simulink model "atrias_boom_nmStand_fullCtrl"  (R2015a)
settings: Solver=ode23t  StartTime=0.0  StopTime=t_end  FixedStep=0.001  MaxStep=1e-3  RelTol=1e-3
InitFcn:
  | addpath('../common/')
  | colors
StartFcn:
  | tic
StopFcn:
  | %stopscript
values from neighbouring files (symbols this model uses):
  A1_notch_f1 = -2*cos(fnotch_f1*sample_time)    [set_control_params.m]
  A2_notch_f1 = 1    [set_control_params.m]
  A_lpf_dtau = 1 + B1_lpf_dtau + B2_lpf_dtau    [set_control_params.m]
  ankle_stiffness = 1/2*pi    (= 1.57079632679)    [mechanical_params.m]
  B1_lpf_dtau = -2*exp(-lpf_damping*fcut_dtau*sample_time)*cos(fcut_dtau*sample_time*sqrt(1-lpf_damping^2))    [set_control_params.m]
  B1_notch_f1 = -2*exp(-notch_damping*fnotch_f1*sample_time)*cos(fnotch_f1*sample_time*sqrt(1-notch_damping^2))    [set_control_params.m]
  B2_lpf_dtau = exp(-2*lpf_damping*fcut_dtau*sample_time)    [set_control_params.m]
  B2_notch_f1 = exp(-2*notch_damping*fnotch_f1*sample_time)    [set_control_params.m]
  b_hmotor = 0    [mechanical_params.m]
  b_leg_spring = 0.075*sqrt(k_leg_spring*0.5*.25^2)    [mechanical_params.m]
  b_rotor = 0*60/(2*pi)*9.725e-5    (= 0)    [mechanical_params.m]
  boom_mount_to_center_diagonal = boom_mount_to_center / cos(pitch_mount_angle)    [mechanical_params.m]    (also in set_control_params.m)
  breakaway_friction = [25 25 25 25]    [mechanical_params.m]
  contactThr = 0.35    [set_control_params.m]
  coulomb_friction = [20 20 20 20]    [mechanical_params.m]
  d_com = (d_hip_com_to_torso_com*m_torso)/(m_torso + num_legs*m_hshaft)    [mechanical_params.m]
  delta_phi_max = 160*pi/180    (= 2.79252680319)    [mechanical_params.m]    (also in set_control_params.m)
  delta_phi_max_buffer = 20*pi/180    (= 0.349065850399)    [set_control_params.m]
  delta_phi_max_dropoff = 2*pi/180    (= 0.0349065850399)    [set_control_params.m]
  delta_phi_min = 25.5*pi/180    (= 0.445058959259)    [mechanical_params.m]    (also in set_control_params.m)
  friction_linear_zone = [0.5 0.5 0.5 0.5].*pi/180    [mechanical_params.m]
  g = 9.803    [mechanical_params.m]    (also in set_control_params.m = 9.81)
  gain_nodes_sea_torque = [0,65,350,700]    [set_control_params.m]
  HIP_MTR_MAX_CONT_TORQUE = HIP_MTR_MAX_CONT_CURRENT*HIP_MOTOR_CONSTANT*HIP_MTR_GEAR_RATIO    (= 86.0016)    [set_control_params.m]
  HIP_MTR_MAX_TORQUE = max_current_hip*Kt_hip*N_h    (= 629.28)    [mechanical_params.m]
  initial_boom_pitch = 0    [mechanical_params.m]
  initial_boom_roll = asin((initial_com_height + boom_mount_to_com + boom_mount_to_center*tan(pitch_mount_angle) - (base_12(2) + yshaft_12(2))) / (l_boom + boom_mount_to_center_diagonal))    [mechanical_params.m]
  initial_boom_yaw = 0    [mechanical_params.m]
  initial_hip_roll = 0*pi/180    (= 0)    [mechanical_params.m]
  initial_winch_angle = -12 * pi/180    (= -0.209439510239)    [mechanical_params.m]
  k_gn = m_total*g/0.01    (= 57041.421916)    [mechanical_params.m]
  k_gt = m_total*g/0.1    (= 5704.1421916)    [mechanical_params.m]
  k_leg_spring = 4118.3    [mechanical_params.m]    (also in set_control_params.m)
  K_notch_f1 = (1+B1_notch_f1+B2_notch_f1)/(1+A1_notch_f1+A2_notch_f1)    [set_control_params.m]
  k_phi = 5000    [mechanical_params.m]
  k_sea = [4118.3 4118.3 4118.3 4118.3]    [set_control_params.m]
  Kb_leg = 0.121    [mechanical_params.m]
  kd_boom_roll_Ctrl = 0    [main_1_nmStand.m]    (also in main_2_nmStand_moveBoom.m)
  kd_lateral = 2*sqrt(kp_lateral*0.8)    [set_control_params.m]
  kd_shin_max = kd_pd_avoid_limits    (= 1000)    [set_control_params.m]
  kd_shin_min = kd_pd_avoid_limits    (= 1000)    [set_control_params.m]
  kd_splay_max = kd_pd_avoid_limits    (= 1000)    [set_control_params.m]
  kd_splay_min = kd_pd_avoid_limits    (= 1000)    [set_control_params.m]
  kd_thigh_max = kd_pd_avoid_limits    (= 1000)    [set_control_params.m]
  kd_thigh_min = kd_pd_avoid_limits    (= 1000)    [set_control_params.m]
  kd_winch = td_winch*kp_winch    (= 989.239577798)    [mechanical_params.m]
  kp_boom_roll_Ctrl = 0    [main_1_nmStand.m]    (also in main_2_nmStand_moveBoom.m)
  kp_lateral = 1000    [set_control_params.m]
  kp_sea_torque = [0.3, 0.3, 6.0, 6.0]    [set_control_params.m]
  kp_shin_max = kp_pd_avoid_limits    (= 5000)    [set_control_params.m]
  kp_shin_min = kp_pd_avoid_limits    (= 5000)    [set_control_params.m]
  kp_splay_max = kp_pd_avoid_limits    (= 5000)    [set_control_params.m]
  kp_splay_min = kp_pd_avoid_limits/10    (= 500)    [set_control_params.m]
  kp_thigh_max = kp_pd_avoid_limits    (= 5000)    [set_control_params.m]
  kp_thigh_min = kp_pd_avoid_limits    (= 5000)    [set_control_params.m]
  kp_winch = winch_gravity_comp/(3*pi/180)    (= 19784.791556)    [mechanical_params.m]
  Kt_leg = 0.121    [mechanical_params.m]
  l_boom = 1.8161    [mechanical_params.m]    (also in set_control_params.m)
  L_leg = 0.102e-3    (= 0.000102)    [mechanical_params.m]
  l_seg = 0.5    [mechanical_params.m]    (also in set_control_params.m)
  l_v = l_seg*cos(min_splay_angle/2)    [set_control_params.m]
  lateral_offset = 0.2    [set_control_params.m]
  lateral_target_angle_right = -6*pi/180    (= -0.10471975512)    [set_control_params.m]
  lateral_transition_force = 150    [set_control_params.m]
  LEG_MTR_MAX_TORQUE = max_current_leg * Kt_leg * N    (= 1210)    [mechanical_params.m]
  loaded_unloaded_torque_threshold = 65*ones(1,4)    [set_control_params.m]
  lowerleg_12 = 0.40    (= 0.4)    [mechanical_params.m]
  m_boom = 4.49    [mechanical_params.m]
  m_fblink = 0.46    [mechanical_params.m]    (also in set_control_params.m)
  m_foot = 0.0857    [mechanical_params.m]
  m_hshaft = 18    [mechanical_params.m]    (also in set_control_params.m = 20)
  m_leg = m_thigh + m_lowerleg + m_shin + m_fblink    (= 2.3438)    [mechanical_params.m]
  m_leg_motor = 18    [set_control_params.m]
  m_lowerleg = 0.4438    [mechanical_params.m]    (also in set_control_params.m)
  m_output_gear = 1e-5    (= 1e-05)    [mechanical_params.m]    (also in set_control_params.m)
  m_rotor = 1e-5    (= 1e-05)    [mechanical_params.m]    (also in set_control_params.m)
  m_shin = 0.75    [mechanical_params.m]    (also in set_control_params.m)
  m_thigh = 0.69    [mechanical_params.m]    (also in set_control_params.m)
  m_torso = 17.5    [mechanical_params.m]    (also in set_control_params.m = 17.9)
  m_total = num_legs*(m_hshaft + m_thigh + m_lowerleg + m_shin + m_fblink + 2*m_gearing) + m_torso    (= 58.18772)    [mechanical_params.m]    (also in set_control_params.m = 62.58772)
  m_virtual_gear = 1e-5    (= 1e-05)    [mechanical_params.m]    (also in set_control_params.m)
  m_yshaft = 12.89    [mechanical_params.m]
  max_current_leg = 200    [mechanical_params.m]
  max_sagittal_loaded_torque = 833    [set_control_params.m]
  max_sagittal_unloaded_torque = 267    [set_control_params.m]
  max_torque_lateral = min(MTR_HIP_MAX_CURRENT, HIP_CURRENT_LIMIT)*HIP_MOTOR_CONSTANT*HIP_MTR_GEAR_RATIO    [set_control_params.m]
  max_voltage_leg = 50    [mechanical_params.m]
  maximum_lateral_angle = 18*pi/180    (= 0.314159265359)    [set_control_params.m]
  min_splay_angle = 45*pi/180    (= 0.785398163397)    [set_control_params.m]
  min_splay_buffer = 1*pi/180    (= 0.0174532925199)    [set_control_params.m]
  min_splay_dropoff = 5*pi/180    (= 0.0872664625997)    [set_control_params.m]
  minimum_lateral_angle = -9.5*pi/180    (= -0.165806278939)    [set_control_params.m]
  mu_hmotor = 0.90    (= 0.9)    [mechanical_params.m]
  mu_motor = 0.85    [mechanical_params.m]
  mu_slide = 0.8    [mechanical_params.m]
  mu_stick = 0.9    [mechanical_params.m]
  N = 50    [mechanical_params.m]
  N_h = r_hip_shaft / r_hip_gearhead    (= 57)    [mechanical_params.m]
  phi_max_collision = -5*pi/180    (= -0.0872664625997)    [mechanical_params.m]
  phi_roll_max = pi + 16*pi/180    (= 3.42084533391)    [mechanical_params.m]
  phi_roll_min = pi - 9*pi/180    (= 2.98451302091)    [mechanical_params.m]
  phi_shin_max = 3*pi/2 + 17.5*pi/180    (= 5.01782159948)    [mechanical_params.m]    (also in set_control_params.m)
  phi_shin_max_buffer = 20*pi/180    (= 0.349065850399)    [set_control_params.m]
  phi_shin_max_dropoff = 2*pi/180    (= 0.0349065850399)    [set_control_params.m]
  phi_shin_min = pi - 45*pi/180    (= 2.35619449019)    [mechanical_params.m]    (also in set_control_params.m)
  phi_shin_min_buffer = 20*pi/180    (= 0.349065850399)    [set_control_params.m]
  phi_shin_min_dropoff = 2*pi/180    (= 0.0349065850399)    [set_control_params.m]
  phi_thigh_max = pi + 45*pi/180    (= 3.92699081699)    [mechanical_params.m]    (also in set_control_params.m)
  phi_thigh_max_buffer = 20*pi/180    (= 0.349065850399)    [set_control_params.m]
  phi_thigh_max_dropoff = 2*pi/180    (= 0.0349065850399)    [set_control_params.m]
  phi_thigh_min = pi/2 - 17.5*pi/180    (= 1.2653637077)    [mechanical_params.m]    (also in set_control_params.m)
  phi_thigh_min_buffer = 20*pi/180    (= 0.349065850399)    [set_control_params.m]
  phi_thigh_min_dropoff = 2*pi/180    (= 0.0349065850399)    [set_control_params.m]
  r_hip_gearhead = 0.009525    [mechanical_params.m]
  r_hip_shaft = 0.542925    [mechanical_params.m]
  R_leg = 0.052    [mechanical_params.m]
  r_rotor = 0.001    [mechanical_params.m]
  r_virtual_gear = N*r_rotor    (= 0.05)    [mechanical_params.m]
  releaseThr = 0.2    [set_control_params.m]
  sample_time = 0.001    [set_control_params.m]
  ... (+19 more)
undefined symbols (not defined in the file or in its folder): A_lpf_velocity, B1_lpf_velocity, B2_lpf_velocity, base_color_d, boom_color_d, c, c_jointstop, CtrlPar_theta0, eref, fblink_color_d, floor_color_d, FmaxBFSH, FmaxGLU, FmaxHAM, FmaxHFL, FmaxRF, FmaxVAS, foot_color_d, FPCtrlPar, hshaft_color_d, j_motor, K, lateral_motor_efficiency, LLCtrlPar, loptBFSH, loptGLU, loptHAM, loptHFL, loptRF, loptVAS, lowerleg_color_d, lslackBFSH, lslackGLU, lslackHAM, lslackHFL, lslackRF, lslackVAS, MidDelay_discrete, Newton, output_sample_time, phi12_max, phi12_min, phi23_max, phi23_min, phimaxRFk, phimaxVAS, phirefBFSH, phirefGLU, phirefHAMh, phirefHAMk, phirefHFL, phirefRFh, phirefRFk, phirefVAS, phiScaleRFk, phiScaleVAS, rad ... (+40)
libraries: sm_lib x210, nesl_utility x140, simulink x58, simulink_extras x26, fl_lib x16, mblibv1 x2, commnoisgen2 x1
(part 13 of 19)

== system atrias_boom_nmStand_fullCtrl/Control/Behavior Control/Virtual Neuromuscular Control/Muscle Layer/L Knee Joint Limits ==
  note: Knee Joint Limits
  phi [rad]1 : Inport
  dphi [rad/s]1 : Inport  Port=2
  Constant : Constant  Value=0
  Gain1 : Gain  Gain=c_jointstop
  Gain5 : Gain  Gain=-1
  Gain6 : Gain  Gain=c_jointstop
  Gain7 : Gain  Gain=1/w_max_jointstop
  Manual Switch : ManualSwitch
  Mux1 : Mux  Inputs=2
  Mux2 : Mux  Inputs=2
  Overextension Torque1 : Fcn  Expr="- u(1)  *  (1-u(2)) * (u(2)<1) * (u(1)>0)"
  Overflexion Torque : Fcn  Expr="- u(1)  *  (1-u(2)) * (u(2)<1) * (u(1)<0)"
  Sum1 : Sum  Inputs=|+-
  Sum2 : Sum  Inputs=|+-
  Sum3 : Sum
  overextension angle1 : Constant  Value=phi12_max
  overflexion angle : Constant  Value=phi12_min
  M_stop [Nm]1 : Outport
  wires:
  Mux2/1 -> Overextension Torque1/1
  Gain6/1 -> Mux2/1
  dphi [rad/s]1/1 -> Gain7/1
  overextension angle1/1 -> Sum1/2
  phi [rad]1/1 -> Sum1/1, Sum2/1
  Sum1/1 -> Gain6/1
  Gain7/1 -> Gain5/1, Mux1/2
  Gain1/1 -> Mux1/1
  Sum2/1 -> Gain1/1
  overflexion angle/1 -> Sum2/2
  Mux1/1 -> Overflexion Torque/1
  Gain5/1 -> Mux2/2
  Overflexion Torque/1 -> Sum3/2
  Overextension Torque1/1 -> Sum3/1
  Sum3/1 -> Manual Switch/1
  Constant/1 -> Manual Switch/2
  Manual Switch/1 -> M_stop [Nm]1/1

== system atrias_boom_nmStand_fullCtrl/Control/Behavior Control/Virtual Neuromuscular Control/Muscle Layer/L Knee Joint Limits1 ==
  note: Knee Joint Limits
  phi [rad]1 : Inport
  dphi [rad/s]1 : Inport  Port=2
  Constant : Constant  Value=0
  Gain1 : Gain  Gain=c_jointstop
  Gain5 : Gain  Gain=-1
  Gain6 : Gain  Gain=c_jointstop
  Gain7 : Gain  Gain=1/w_max_jointstop
  Manual Switch : ManualSwitch
  Mux1 : Mux  Inputs=2
  Mux2 : Mux  Inputs=2
  Overextension Torque1 : Fcn  Expr="- u(1)  *  (1-u(2)) * (u(2)<1) * (u(1)>0)"
  Overflexion Torque : Fcn  Expr="- u(1)  *  (1-u(2)) * (u(2)<1) * (u(1)<0)"
  Sum1 : Sum  Inputs=|+-
  Sum2 : Sum  Inputs=|+-
  Sum3 : Sum
  overextension angle1 : Constant  Value=phi12_max
  overflexion angle : Constant  Value=phi12_min
  M_stop [Nm]1 : Outport
  wires:
  Mux2/1 -> Overextension Torque1/1
  Gain6/1 -> Mux2/1
  dphi [rad/s]1/1 -> Gain7/1
  overextension angle1/1 -> Sum1/2
  phi [rad]1/1 -> Sum1/1, Sum2/1
  Sum1/1 -> Gain6/1
  Gain7/1 -> Gain5/1, Mux1/2
  Gain1/1 -> Mux1/1
  Sum2/1 -> Gain1/1
  overflexion angle/1 -> Sum2/2
  Mux1/1 -> Overflexion Torque/1
  Gain5/1 -> Mux2/2
  Overflexion Torque/1 -> Sum3/2
  Overextension Torque1/1 -> Sum3/1
  Sum3/1 -> Manual Switch/1
  Constant/1 -> Manual Switch/2
  Manual Switch/1 -> M_stop [Nm]1/1

== system atrias_boom_nmStand_fullCtrl/Control/Behavior Control/Virtual Neuromuscular Control/Muscle Layer/RF ==
  note: Rectus Femoris Muscle-Tendon Dynamics
  note: Excitation Contraction Coupling
  STIM : Inport
  lmtc [m] : Inport  Port=2
  1 : Product  Inputs=**  SaturateOnIntegerOverflow=on  InputSameDT=on  OutDataTypeStr=Inherit: Same as first input
  1/lslack : Gain  Gain=1/lslackRF  SaturateOnIntegerOverflow=on  OutDataTypeStr=Inherit: Same as input  ParamDataTypeStr=Inherit: Same as input
  BE force-length relation : Subsystem
  CE force-length relation : Subsystem
  CE inverse force-velocity relation : Subsystem
  Constant : Constant  Value=lslackRF
  ECC TransferFcn : simulink_extras/Additional Linear/Transfer Fcn (with initial outputs)  N=[1]  D="[tau  1]"  Y0=preA  U0=0
      settings: AttributesFormatString=pre-activation: %<Y0>
  Fmax : Gain  Gain=FmaxRF  SaturateOnIntegerOverflow=on  OutDataTypeStr=Inherit: Same as input  ParamDataTypeStr=Inherit: Same as input
  Fv = Fse / (A*Fce) : Product  Inputs=*/  SaturateOnIntegerOverflow=on  InputSameDT=on  OutDataTypeStr=Inherit: Same as first input
  Integrator : Integrator  InitialConditionSource=external  LowerSaturationLimit=0.05
  PE force-length relation : Subsystem
  SE force-length relation : Subsystem
  Saturation : Saturate  UpperLimit=1  LowerLimit=0.01
  Sum : Sum  Inputs=|+-  SaturateOnIntegerOverflow=on  InputSameDT=on  OutDataTypeStr=Inherit: Same as first input
  Sum2 : Sum  Inputs=|-+  SaturateOnIntegerOverflow=on  InputSameDT=on  OutDataTypeStr=Inherit: Same as first input
  Sum3 : Sum  SaturateOnIntegerOverflow=on  InputSameDT=on  OutDataTypeStr=Inherit: Same as first input
  Sum4 : Sum  SaturateOnIntegerOverflow=on  InputSameDT=on  OutDataTypeStr=Inherit: Same as first input
  lce/lopt : Gain  Gain=1/loptRF  SaturateOnIntegerOverflow=on  OutDataTypeStr=Inherit: Same as input  ParamDataTypeStr=Inherit: Same as input
  vmax*lopt : Gain  Gain=vmaxRF*loptRF  SaturateOnIntegerOverflow=on  OutDataTypeStr=Inherit: Same as input  ParamDataTypeStr=Inherit: Same as input
  Fmtc : Outport  InitialOutput=0
  Lce : Outport  Port=2  InitialOutput=0
  Vce : Outport  Port=3  InitialOutput=0
  A : Outport  Port=4  InitialOutput=0
  wires:
  Integrator/1 -> Sum/2, lce/lopt/1, Lce/1  "lce"
  Sum/1 -> 1/lslack/1  "lse"
  lce/lopt/1 -> CE force-length relation/1(lce [lopt]), BE force-length relation/1(lce [lopt]), PE force-length relation/1(lce [lopt])
  Fv = Fse / (A*Fce)/1 -> CE inverse force-velocity relation/1(Fv[Fmax])  "fv"
  vmax*lopt/1 -> Integrator/1, Vce/1  "vce"
  lmtc [m]/1 -> Sum2/2, Sum/1  "lmtc"
  Fmax/1 -> Fmtc/1  "Fmtc"
  1/lslack/1 -> SE force-length relation/1(lse [lslack])
  SE force-length relation/1(fse [Fmax]) -> Fmax/1, Sum4/1
  Sum2/1 -> Integrator/2
  Constant/1 -> Sum2/1
  CE force-length relation/1(fce [Fmax]) -> 1/1
  Sum4/1 -> Fv = Fse / (A*Fce)/1
  PE force-length relation/1(fpe [Fmax]) -> Sum3/1
  1/1 -> Sum3/2
  BE force-length relation/1(fbe [Fmax]) -> Sum4/2
  Sum3/1 -> Fv = Fse / (A*Fce)/2
  CE inverse force-velocity relation/1(v[vmax]) -> vmax*lopt/1
  STIM/1 -> ECC TransferFcn/1
  ECC TransferFcn/1 -> Saturation/1
  Saturation/1 -> 1/2, A/1

== system atrias_boom_nmStand_fullCtrl/Control/Behavior Control/Virtual Neuromuscular Control/Muscle Layer/RF Link ==
  note: RF Attachment
  phi34 [rad] : Inport
  phi23 [rad] : Inport  Port=2
  Constant1 : Constant  Value=phimaxRFk
  Constant2 : Constant  Value=phirefRFk
  Constant3 : Constant  Value=rRFh
  Constant4 : Constant  Value=lslackRF+loptRF
  Constant5 : Constant  Value=phirefRFh
  Demux : Demux  Outputs=2
  Display : Display
  Gain1 : Gain  Gain=rRFkmax
  Gain2 : Gain  Gain=rhoRFh
  Gain3 : Gain  Gain=phiScaleRFk
  Gain4 : Gain  Gain=rhoRFk/phiScaleRFk
  Gain5 : Gain  Gain=phiScaleRFk
  Mux : Mux  Inputs=2
  Product : Product  RndMeth=Zero
  Sum1 : Sum  Inputs=-+
  Sum2 : Sum  Inputs=|+-
  Sum3 : Sum  Inputs=-+|
  Sum4 : Sum  Inputs=|+-
  Sum5 : Sum  Inputs=++-
  length change term : Trigonometry
  offset correction term : Trigonometry
  variable lever term : Trigonometry  Operator=cos
  lmtu [m] : Outport
  lever34 [m] : Outport  Port=2
  lever23 [m] : Outport  Port=3
  wires:
  Sum5/1 -> Display/1, lmtu [m]/1
  Constant4/1 -> Sum5/2
  Gain4/1 -> Sum5/3
  Gain2/1 -> Sum5/1
  phi34 [rad]/1 -> Sum4/1
  Constant5/1 -> Sum4/2
  Sum4/1 -> Product/1
  Constant3/1 -> Product/2, lever34 [m]/1
  Product/1 -> Gain2/1
  phi23 [rad]/1 -> Sum3/2
  Sum3/1 -> Gain3/1
  Constant1/1 -> Sum3/1, Sum2/2
  Sum2/1 -> Gain5/1
  Constant2/1 -> Sum2/1
  length change term/1 -> Sum1/2
  offset correction term/1 -> Sum1/1
  Sum1/1 -> Mux/1
  variable lever term/1 -> Mux/2
  Mux/1 -> Gain1/1
  Gain1/1 -> Demux/1
  Demux/2 -> lever23 [m]/1
  Demux/1 -> Gain4/1
  Gain3/1 -> variable lever term/1, length change term/1
  Gain5/1 -> offset correction term/1

== system atrias_boom_nmStand_fullCtrl/Control/Behavior Control/Virtual Neuromuscular Control/Muscle Layer/RF Link1 ==
  note: RF Attachment
  phi34 [rad] : Inport
  phi23 [rad] : Inport  Port=2
  Constant1 : Constant  Value=phimaxRFk
  Constant2 : Constant  Value=phirefRFk
  Constant3 : Constant  Value=rRFh
  Constant4 : Constant  Value=lslackRF+loptRF
  Constant5 : Constant  Value=phirefRFh
  Demux : Demux  Outputs=2
  Gain1 : Gain  Gain=rRFkmax
  Gain2 : Gain  Gain=rhoRFh
  Gain3 : Gain  Gain=phiScaleRFk
  Gain4 : Gain  Gain=rhoRFk/phiScaleRFk
  Gain5 : Gain  Gain=phiScaleRFk
  Mux : Mux  Inputs=2
  Product : Product  RndMeth=Zero
  Sum1 : Sum  Inputs=-+
  Sum2 : Sum  Inputs=|+-
  Sum3 : Sum  Inputs=-+|
  Sum4 : Sum  Inputs=|+-
  Sum5 : Sum  Inputs=++-
  length change term : Trigonometry
  offset correction term : Trigonometry
  variable lever term : Trigonometry  Operator=cos
  lmtu [m] : Outport
  lever34 [m] : Outport  Port=2
  lever23 [m] : Outport  Port=3
  wires:
  Sum5/1 -> lmtu [m]/1
  Constant4/1 -> Sum5/2
  Gain4/1 -> Sum5/3
  Gain2/1 -> Sum5/1
  phi34 [rad]/1 -> Sum4/1
  Constant5/1 -> Sum4/2
  Sum4/1 -> Product/1
  Constant3/1 -> Product/2, lever34 [m]/1
  Product/1 -> Gain2/1
  phi23 [rad]/1 -> Sum3/2
  Sum3/1 -> Gain3/1
  Constant1/1 -> Sum3/1, Sum2/2
  Sum2/1 -> Gain5/1
  Constant2/1 -> Sum2/1
  length change term/1 -> Sum1/2
  offset correction term/1 -> Sum1/1
  Sum1/1 -> Mux/1
  variable lever term/1 -> Mux/2
  Mux/1 -> Gain1/1
  Gain1/1 -> Demux/1
  Demux/2 -> lever23 [m]/1
  Demux/1 -> Gain4/1
  Gain3/1 -> variable lever term/1, length change term/1
  Gain5/1 -> offset correction term/1

== system atrias_boom_nmStand_fullCtrl/Control/Behavior Control/Virtual Neuromuscular Control/Muscle Layer/RF1 ==
  note: Rectus Femoris Muscle-Tendon Dynamics
  note: Excitation Contraction Coupling
  STIM : Inport
  lmtc [m] : Inport  Port=2
  1 : Product  Inputs=**  SaturateOnIntegerOverflow=on  InputSameDT=on  OutDataTypeStr=Inherit: Same as first input
  1/lslack : Gain  Gain=1/lslackRF  SaturateOnIntegerOverflow=on  OutDataTypeStr=Inherit: Same as input  ParamDataTypeStr=Inherit: Same as input
  BE force-length relation : Subsystem
  CE force-length relation : Subsystem
  CE inverse force-velocity relation : Subsystem
  Constant : Constant  Value=lslackRF
  ECC TransferFcn : simulink_extras/Additional Linear/Transfer Fcn (with initial outputs)  N=[1]  D="[tau  1]"  Y0=preA  U0=0
      settings: AttributesFormatString=pre-activation: %<Y0>
  Fmax : Gain  Gain=FmaxRF  SaturateOnIntegerOverflow=on  OutDataTypeStr=Inherit: Same as input  ParamDataTypeStr=Inherit: Same as input
  Fv = Fse / (A*Fce) : Product  Inputs=*/  SaturateOnIntegerOverflow=on  InputSameDT=on  OutDataTypeStr=Inherit: Same as first input
  Integrator : Integrator  InitialConditionSource=external  LowerSaturationLimit=0.05
  PE force-length relation : Subsystem
  SE force-length relation : Subsystem
  Saturation : Saturate  UpperLimit=1  LowerLimit=0.01
  Sum : Sum  Inputs=|+-  SaturateOnIntegerOverflow=on  InputSameDT=on  OutDataTypeStr=Inherit: Same as first input
  Sum2 : Sum  Inputs=|-+  SaturateOnIntegerOverflow=on  InputSameDT=on  OutDataTypeStr=Inherit: Same as first input
  Sum3 : Sum  SaturateOnIntegerOverflow=on  InputSameDT=on  OutDataTypeStr=Inherit: Same as first input
  Sum4 : Sum  SaturateOnIntegerOverflow=on  InputSameDT=on  OutDataTypeStr=Inherit: Same as first input
  lce/lopt : Gain  Gain=1/loptRF  SaturateOnIntegerOverflow=on  OutDataTypeStr=Inherit: Same as input  ParamDataTypeStr=Inherit: Same as input
  vmax*lopt : Gain  Gain=vmaxRF*loptRF  SaturateOnIntegerOverflow=on  OutDataTypeStr=Inherit: Same as input  ParamDataTypeStr=Inherit: Same as input
  Fmtc : Outport  InitialOutput=0
  Lce : Outport  Port=2  InitialOutput=0
  Vce : Outport  Port=3  InitialOutput=0
  A : Outport  Port=4  InitialOutput=0
  wires:
  Integrator/1 -> Sum/2, lce/lopt/1, Lce/1  "lce"
  Sum/1 -> 1/lslack/1  "lse"
  lce/lopt/1 -> CE force-length relation/1(lce [lopt]), BE force-length relation/1(lce [lopt]), PE force-length relation/1(lce [lopt])
  Fv = Fse / (A*Fce)/1 -> CE inverse force-velocity relation/1(Fv[Fmax])  "fv"
  vmax*lopt/1 -> Integrator/1, Vce/1  "vce"
  lmtc [m]/1 -> Sum2/2, Sum/1  "lmtc"
  Fmax/1 -> Fmtc/1  "Fmtc"
  1/lslack/1 -> SE force-length relation/1(lse [lslack])
  SE force-length relation/1(fse [Fmax]) -> Fmax/1, Sum4/1
  Sum2/1 -> Integrator/2
  Constant/1 -> Sum2/1
  CE force-length relation/1(fce [Fmax]) -> 1/1
  Sum4/1 -> Fv = Fse / (A*Fce)/1
  PE force-length relation/1(fpe [Fmax]) -> Sum3/1
  1/1 -> Sum3/2
  BE force-length relation/1(fbe [Fmax]) -> Sum4/2
  Sum3/1 -> Fv = Fse / (A*Fce)/2
  CE inverse force-velocity relation/1(v[vmax]) -> vmax*lopt/1
  STIM/1 -> ECC TransferFcn/1
  ECC TransferFcn/1 -> Saturation/1
  Saturation/1 -> 1/2, A/1

== system atrias_boom_nmStand_fullCtrl/Control/Behavior Control/Virtual Neuromuscular Control/Muscle Layer/VAS ==
  note: VASTI Muscle-Tendon Dynamics
  note: Excitation Contraction Coupling
  STIM : Inport
  lmtc [m] : Inport  Port=2
  1 : Product  Inputs=**  SaturateOnIntegerOverflow=on  InputSameDT=on  OutDataTypeStr=Inherit: Same as first input
  1/lslack : Gain  Gain=1/lslackVAS  SaturateOnIntegerOverflow=on  OutDataTypeStr=Inherit: Same as input  ParamDataTypeStr=Inherit: Same as input
  BE force-length relation : Subsystem
  CE force-length relation : Subsystem
  CE inverse force-velocity relation : Subsystem
  Constant : Constant  Value=lslackVAS
  ECC TransferFcn : simulink_extras/Additional Linear/Transfer Fcn (with initial outputs)  N=[1]  D="[tau  1]"  Y0=preA  U0=0
      settings: AttributesFormatString=pre-activation: %<Y0>
  Fmax : Gain  Gain=FmaxVAS  SaturateOnIntegerOverflow=on  OutDataTypeStr=Inherit: Same as input  ParamDataTypeStr=Inherit: Same as input
  Fv = Fse / (A*Fce) : Product  Inputs=*/  SaturateOnIntegerOverflow=on  InputSameDT=on  OutDataTypeStr=Inherit: Same as first input
  Integrator : Integrator  InitialConditionSource=external  LowerSaturationLimit=0.05
  PE force-length relation : Subsystem
  SE force-length relation : Subsystem
  Saturation : Saturate  UpperLimit=1  LowerLimit=0.01
  Sum : Sum  Inputs=|+-  SaturateOnIntegerOverflow=on  InputSameDT=on  OutDataTypeStr=Inherit: Same as first input
  Sum2 : Sum  Inputs=|-+  SaturateOnIntegerOverflow=on  InputSameDT=on  OutDataTypeStr=Inherit: Same as first input
  Sum3 : Sum  SaturateOnIntegerOverflow=on  InputSameDT=on  OutDataTypeStr=Inherit: Same as first input
  Sum4 : Sum  SaturateOnIntegerOverflow=on  InputSameDT=on  OutDataTypeStr=Inherit: Same as first input
  lce/lopt : Gain  Gain=1/loptVAS  SaturateOnIntegerOverflow=on  OutDataTypeStr=Inherit: Same as input  ParamDataTypeStr=Inherit: Same as input
  vmax*lopt : Gain  Gain=vmaxVAS*loptVAS  SaturateOnIntegerOverflow=on  OutDataTypeStr=Inherit: Same as input  ParamDataTypeStr=Inherit: Same as input
  Fmtc : Outport  InitialOutput=0
  Lce : Outport  Port=2  InitialOutput=0
  Vce : Outport  Port=3  InitialOutput=0
  A : Outport  Port=4  InitialOutput=0
  wires:
  Integrator/1 -> Sum/2, lce/lopt/1, Lce/1  "lce"
  Sum/1 -> 1/lslack/1  "lse"
  lce/lopt/1 -> CE force-length relation/1(lce [lopt]), BE force-length relation/1(lce [lopt]), PE force-length relation/1(lce [lopt])
  Fv = Fse / (A*Fce)/1 -> CE inverse force-velocity relation/1(Fv[Fmax])  "fv"
  vmax*lopt/1 -> Integrator/1, Vce/1  "vce"
  lmtc [m]/1 -> Sum2/2, Sum/1  "lmtc"
  Fmax/1 -> Fmtc/1  "Fmtc"
  1/lslack/1 -> SE force-length relation/1(lse [lslack])
  SE force-length relation/1(fse [Fmax]) -> Fmax/1, Sum4/1
  Sum2/1 -> Integrator/2
  Constant/1 -> Sum2/1
  CE force-length relation/1(fce [Fmax]) -> 1/1
  Sum4/1 -> Fv = Fse / (A*Fce)/1
  PE force-length relation/1(fpe [Fmax]) -> Sum3/1
  1/1 -> Sum3/2
  BE force-length relation/1(fbe [Fmax]) -> Sum4/2
  Sum3/1 -> Fv = Fse / (A*Fce)/2
  CE inverse force-velocity relation/1(v[vmax]) -> vmax*lopt/1
  STIM/1 -> ECC TransferFcn/1
  ECC TransferFcn/1 -> Saturation/1
  Saturation/1 -> 1/2, A/1

== system atrias_boom_nmStand_fullCtrl/Control/Behavior Control/Virtual Neuromuscular Control/Muscle Layer/VAS Link ==
  note: Muscle Length and Moment Arm
  phi23 [rad] : Inport
  Constant : Constant  Value=lslackVAS+loptVAS
  Constant1 : Constant  Value=phimaxVAS
  Constant2 : Constant  Value=phirefVAS
  Demux : Demux  Outputs=2
  Gain1 : Gain  Gain=rVASmax
  Gain3 : Gain  Gain=phiScaleVAS
  Gain4 : Gain  Gain=rhoVAS/phiScaleVAS
  Gain5 : Gain  Gain=phiScaleVAS
  Mux : Mux  Inputs=2
  Sum1 : Sum  Inputs=-+
  Sum2 : Sum  Inputs=|+-
  Sum3 : Sum  Inputs=-+|
  Sum5 : Sum  Inputs=|+-
  length change term : Trigonometry
  offset correction term : Trigonometry
  variable lever term : Trigonometry  Operator=cos
  lmtu [m] : Outport
  lever [m] : Outport  Port=2
  wires:
  Constant/1 -> Sum5/1
  Sum5/1 -> lmtu [m]/1
  phi23 [rad]/1 -> Sum3/2
  Sum3/1 -> Gain3/1
  Constant1/1 -> Sum3/1, Sum2/2
  Sum2/1 -> Gain5/1
  Constant2/1 -> Sum2/1
  length change term/1 -> Sum1/2
  offset correction term/1 -> Sum1/1
  Sum1/1 -> Mux/1
  variable lever term/1 -> Mux/2
  Mux/1 -> Gain1/1
  Gain1/1 -> Demux/1
  Demux/2 -> lever [m]/1
  Demux/1 -> Gain4/1
  Gain3/1 -> variable lever term/1, length change term/1
  Gain5/1 -> offset correction term/1
  Gain4/1 -> Sum5/2

== system atrias_boom_nmStand_fullCtrl/Control/Behavior Control/Virtual Neuromuscular Control/Muscle Layer/VAS Link1 ==
  note: Muscle Length and Moment Arm
  phi23 [rad] : Inport
  Constant : Constant  Value=lslackVAS+loptVAS
  Constant1 : Constant  Value=phimaxVAS
  Constant2 : Constant  Value=phirefVAS
  Demux : Demux  Outputs=2
  Gain1 : Gain  Gain=rVASmax
  Gain3 : Gain  Gain=phiScaleVAS
  Gain4 : Gain  Gain=rhoVAS/phiScaleVAS
  Gain5 : Gain  Gain=phiScaleVAS
  Mux : Mux  Inputs=2
  Sum1 : Sum  Inputs=-+
  Sum2 : Sum  Inputs=|+-
  Sum3 : Sum  Inputs=-+|
  Sum5 : Sum  Inputs=|+-
  length change term : Trigonometry
  offset correction term : Trigonometry
  variable lever term : Trigonometry  Operator=cos
  lmtu [m] : Outport
  lever [m] : Outport  Port=2
  wires:
  Constant/1 -> Sum5/1
  Sum5/1 -> lmtu [m]/1
  phi23 [rad]/1 -> Sum3/2
  Sum3/1 -> Gain3/1
  Constant1/1 -> Sum3/1, Sum2/2
  Sum2/1 -> Gain5/1
  Constant2/1 -> Sum2/1
  length change term/1 -> Sum1/2
  offset correction term/1 -> Sum1/1
  Sum1/1 -> Mux/1
  variable lever term/1 -> Mux/2
  Mux/1 -> Gain1/1
  Gain1/1 -> Demux/1
  Demux/2 -> lever [m]/1
  Demux/1 -> Gain4/1
  Gain3/1 -> variable lever term/1, length change term/1
  Gain5/1 -> offset correction term/1
  Gain4/1 -> Sum5/2

== system atrias_boom_nmStand_fullCtrl/Control/Behavior Control/Virtual Neuromuscular Control/Muscle Layer/VAS1 ==
  note: VASTI Muscle-Tendon Dynamics
  note: Excitation Contraction Coupling
  STIM : Inport
  lmtc [m] : Inport  Port=2
  1 : Product  Inputs=**  SaturateOnIntegerOverflow=on  InputSameDT=on  OutDataTypeStr=Inherit: Same as first input
  1/lslack : Gain  Gain=1/lslackVAS  SaturateOnIntegerOverflow=on  OutDataTypeStr=Inherit: Same as input  ParamDataTypeStr=Inherit: Same as input
  BE force-length relation : Subsystem
  CE force-length relation : Subsystem
  CE inverse force-velocity relation : Subsystem
  Constant : Constant  Value=lslackVAS
  ECC TransferFcn : simulink_extras/Additional Linear/Transfer Fcn (with initial outputs)  N=[1]  D="[tau  1]"  Y0=preA  U0=0
      settings: AttributesFormatString=pre-activation: %<Y0>
  Fmax : Gain  Gain=FmaxVAS  SaturateOnIntegerOverflow=on  OutDataTypeStr=Inherit: Same as input  ParamDataTypeStr=Inherit: Same as input
  Fv = Fse / (A*Fce) : Product  Inputs=*/  SaturateOnIntegerOverflow=on  InputSameDT=on  OutDataTypeStr=Inherit: Same as first input
  Integrator : Integrator  InitialConditionSource=external  LowerSaturationLimit=0.05
  PE force-length relation : Subsystem
  SE force-length relation : Subsystem
  Saturation : Saturate  UpperLimit=1  LowerLimit=0.01
  Sum : Sum  Inputs=|+-  SaturateOnIntegerOverflow=on  InputSameDT=on  OutDataTypeStr=Inherit: Same as first input
  Sum2 : Sum  Inputs=|-+  SaturateOnIntegerOverflow=on  InputSameDT=on  OutDataTypeStr=Inherit: Same as first input
  Sum3 : Sum  SaturateOnIntegerOverflow=on  InputSameDT=on  OutDataTypeStr=Inherit: Same as first input
  Sum4 : Sum  SaturateOnIntegerOverflow=on  InputSameDT=on  OutDataTypeStr=Inherit: Same as first input
  lce/lopt : Gain  Gain=1/loptVAS  SaturateOnIntegerOverflow=on  OutDataTypeStr=Inherit: Same as input  ParamDataTypeStr=Inherit: Same as input
  vmax*lopt : Gain  Gain=vmaxVAS*loptVAS  SaturateOnIntegerOverflow=on  OutDataTypeStr=Inherit: Same as input  ParamDataTypeStr=Inherit: Same as input
  Fmtc : Outport  InitialOutput=0
  Lce : Outport  Port=2  InitialOutput=0
  Vce : Outport  Port=3  InitialOutput=0
  A : Outport  Port=4  InitialOutput=0
  wires:
  Integrator/1 -> Sum/2, lce/lopt/1, Lce/1  "lce"
  Sum/1 -> 1/lslack/1  "lse"
  lce/lopt/1 -> CE force-length relation/1(lce [lopt]), BE force-length relation/1(lce [lopt]), PE force-length relation/1(lce [lopt])
  Fv = Fse / (A*Fce)/1 -> CE inverse force-velocity relation/1(Fv[Fmax])  "fv"
  vmax*lopt/1 -> Integrator/1, Vce/1  "vce"
  lmtc [m]/1 -> Sum2/2, Sum/1  "lmtc"
  Fmax/1 -> Fmtc/1  "Fmtc"
  1/lslack/1 -> SE force-length relation/1(lse [lslack])
  SE force-length relation/1(fse [Fmax]) -> Fmax/1, Sum4/1
  Sum2/1 -> Integrator/2
  Constant/1 -> Sum2/1
  CE force-length relation/1(fce [Fmax]) -> 1/1
  Sum4/1 -> Fv = Fse / (A*Fce)/1
  PE force-length relation/1(fpe [Fmax]) -> Sum3/1
  1/1 -> Sum3/2
  BE force-length relation/1(fbe [Fmax]) -> Sum4/2
  Sum3/1 -> Fv = Fse / (A*Fce)/2
  CE inverse force-velocity relation/1(v[vmax]) -> vmax*lopt/1
  STIM/1 -> ECC TransferFcn/1
  ECC TransferFcn/1 -> Saturation/1
  Saturation/1 -> 1/2, A/1

== system atrias_boom_nmStand_fullCtrl/Control/Behavior Control/Virtual Neuromuscular Control/Neural Control Layer/L Stance Phase (sagittal) ==
  note: M4: compensate swing leg
  note: M3: balance trunk
  note: M2: prevent knee overextension
  note: M1: realize compliant leg
  note: 0: Prestimulations
  note: Left Stance Phase Control
  CtrlPar : Inport
  theta_tgt [rad] : Inport  Port=2
  theta dtheta [rad rad/s] : Inport  Port=3
  CStim_HSw : Inport  Port=4
  FmVAS : Inport  Port=5
  LceBFSH : Inport  Port=6
  Enable : EnablePort  StatesWhenEnabling=reset  ZeroCross=off
  Demux1 : Demux  Outputs=5
  Demux2 : Demux
  Demux4 : Demux  Outputs=6
  Demux5 : Demux  Outputs=5
  Demux7 : Demux  Outputs=2
  Divide{4..6,8..9,12..13,15,17,19..22} (13 alike) : Product
  Gain : Gain  Gain=-1
  Gain2 : Gain  Gain=-1
  Gain3 : Gain  Gain=-1
  Mux1 : Mux  Inputs=3
  Mux2 : Mux  Inputs=2
  Mux3 : Mux  Inputs=3
  Sum1 : Sum  Inputs=-+|  SaturateOnIntegerOverflow=on  InputSameDT=on  OutDataTypeStr=Inherit: Same as first input
  Sum{2,7..8,11} (4 alike) : Sum  Inputs=|++  SaturateOnIntegerOverflow=on  InputSameDT=on  OutDataTypeStr=Inherit: Same as first input
  Sum3 : Sum  Inputs=-+|  SaturateOnIntegerOverflow=on  InputSameDT=on  OutDataTypeStr=Inherit: Same as first input
  Sum4 : Sum  Inputs=-+|  SaturateOnIntegerOverflow=on  InputSameDT=on  OutDataTypeStr=Inherit: Same as first input
  Terminator : Terminator
  Terminator1 : Terminator
  parStPreS : Selector  InputPortWidth=St_i  Indices=parSt_PreS_i
  parSt_M1 : Selector  InputPortWidth=St_i  Indices=parSt_M1_i
  parSt_M2 : Selector  InputPortWidth=St_i  Indices=parSt_M2_i
  parSt_M3 : Selector  InputPortWidth=St_i  Indices=parSt_M3_i
  parSt_M4 : Selector  InputPortWidth=St_i  Indices=parSt_M4_i
  positive half{1..4,6} (5 alike) : Saturate  UpperLimit=inf  LowerLimit=0  ZeroCross=off
  S_St_0 : Outport  OutputWhenDisabled=reset  InitialOutput=0
  S_M1 [VAS] : Outport  Port=2  OutputWhenDisabled=reset  InitialOutput=0
  S_M2 [VAS BFSH] : Outport  Port=3  OutputWhenDisabled=reset  InitialOutput=0
  S_M3 [HFL GLU HAM] : Outport  Port=4  OutputWhenDisabled=reset  InitialOutput=0
  S_M4 [HFL GLU HAM] : Outport  Port=5  OutputWhenDisabled=reset  InitialOutput=0
  wires:
  Demux4/6 -> Terminator1/1
  Demux4/5 -> Terminator/1
  Divide9/1 -> Sum11/2
  Sum11/1 -> Divide21/1, Mux3/2  "GLU"
  Divide12/1 -> Sum11/1
  Divide17/1 -> Sum7/2
  Sum7/1 -> Mux3/1  "HFL"
  Divide22/1 -> Sum7/1
  Demux1/4 -> Divide9/1  "SGainCRF_GLU"
  Demux1/2 -> Divide17/1  "SGainCHAM_HFL"
  Demux4/4 -> Divide9/2  "Stim_CRF"
  Demux4/3 -> Divide17/2  "Stim_CHAM"
  Divide21/1 -> Mux3/3  "HAM"
  Demux1/5 -> Divide21/2  "SGainGLU_HAM"
  Mux3/1 -> S_M4 [HFL GLU HAM]/1
  Demux4/2 -> Divide22/2  "Stim_CGLU"
  Demux4/1 -> Divide12/2  "Stim_CHFL"
  CStim_HSw/1 -> Demux4/1
  Demux1/3 -> Divide12/1  "SGainCHFL_GLU"
  Demux1/1 -> Divide22/1  "SGainCGLU_HFL"
  parSt_M4/1 -> Demux1/1
  positive half6/1 -> Mux1/3
  positive half2/1 -> Mux1/2
  positive half1/1 -> Mux1/1
  theta_tgt [rad]/1 -> Sum1/1
  Divide6/1 -> positive half6/1  "HAM"
  Demux5/5 -> Divide6/2  "SGainGLU_HAM"
  Mux1/1 -> S_M3 [HFL GLU HAM]/1
  Sum8/1 -> positive half2/1, Divide6/1  "GLU"
  Sum2/1 -> positive half1/1  "HFL"
  Divide5/1 -> Sum8/2
  Divide4/1 -> Sum8/1
  Divide20/1 -> Sum2/2
  Divide19/1 -> Sum2/1
  Gain3/1 -> Divide20/1
  Gain2/1 -> Divide19/1
  Sum1/1 -> Divide4/1, Gain2/1
  Demux7/2 -> Divide5/1, Gain3/1  "dtheta"
  Demux7/1 -> Sum1/2  "theta"
  theta dtheta [rad rad/s]/1 -> Demux7/1
  Demux5/4 -> Divide5/2  "GainDTh_GLU"
  Demux5/3 -> Divide4/2  "GainTh_GLU"
  Demux5/2 -> Divide20/2  "GainDTh_HFL"
  Demux5/1 -> Divide19/2  "GainTh_HFL"
  parSt_M3/1 -> Demux5/1
  Mux2/1 -> S_M2 [VAS BFSH]/1
  LceBFSH/1 -> Sum4/2, Sum3/2
  Demux2/3 -> Sum4/1  "loff_BFSH"
  positive half4/1 -> Divide13/1
  Sum4/1 -> positive half4/1
  Gain/1 -> Mux2/1  "VAS"
  Divide13/1 -> Mux2/2  "BFSH"
  Divide15/1 -> Gain/1
  Demux2/1 -> Sum3/1  "loff_BFSH_VAS"
  positive half3/1 -> Divide15/1
  Demux2/4 -> Divide13/2  "LGain_BFSH"
  Demux2/2 -> Divide15/2  "LGainBFSH_VAS"
  Sum3/1 -> positive half3/1
  parSt_M2/1 -> Demux2/1
  FmVAS/1 -> Divide8/2
  Divide8/1 -> S_M1 [VAS]/1  "VAS"
  parSt_M1/1 -> Divide8/1  "FGain_VAS"
  parStPreS/1 -> S_St_0/1
  CtrlPar/1 -> parSt_M1/1, parSt_M2/1, parSt_M4/1, parSt_M3/1, parStPreS/1

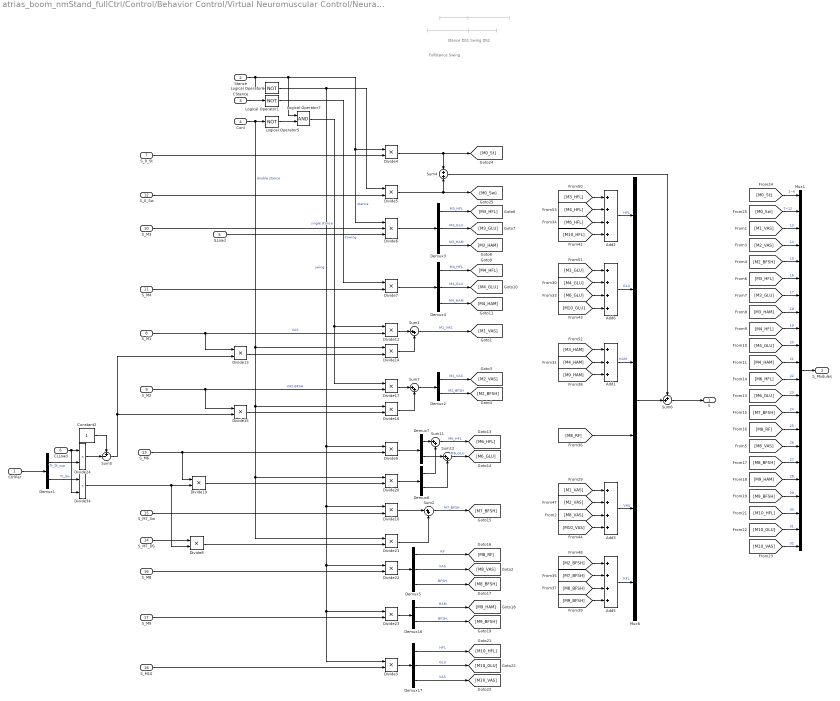
== system atrias_boom_nmStand_fullCtrl/Control/Behavior Control/Virtual Neuromuscular Control/Neural Control Layer/L Stance, Swing, Trans (sagittal) ==
  note: |--------------------|------------------------------|
  note: |------------------------------|--------------------|
  note: FullStance Swing
  note: Stance DS1 Swing DS2
  CtrlPar : Inport
  Stance : Inport  Port=2
  CStance : Inport  Port=3
  ConI : Inport  Port=4
  ILLoad : Inport  Port=5
  CLLoad : Inport  Port=6
  S_0_St : Inport  Port=7
  S_M1 : Inport  Port=8
  S_M2 : Inport  Port=9
  S_M3 : Inport  Port=10
  S_M4 : Inport  Port=11
  S_0_Sw : Inport  Port=12
  S_M6 : Inport  Port=13
  S_M7_DS : Inport  Port=14
  S_M7_Sw : Inport  Port=15
  S_M8 : Inport  Port=16
  S_M9 : Inport  Port=17
  S_M10 : Inport  Port=18
  Add1 : Sum  Inputs=3
  Add{2..3,5..6} (4 alike) : Sum  Inputs=4
  Constant2 : Constant
  Demux{1..2,6..7,16} (5 alike) : Demux  Outputs=2
  Demux{3..5,17} (4 alike) : Demux  Outputs=3
  Divide{3..5,7..10,12..17,19..24,34} (20 alike) : Product
  Divide6 : Product  Inputs=3
  Logical Operator1 : Logic  Operator=NOT  AllPortsSameDT=off  OutDataTypeStr=boolean
  Logical Operator5 : Logic  Operator=NOT  AllPortsSameDT=off  OutDataTypeStr=boolean
  Logical Operator6 : Logic  Operator=NOT  AllPortsSameDT=off  OutDataTypeStr=boolean
  Logical Operator7 : Logic  AllPortsSameDT=off  OutDataTypeStr=boolean
  Mux1 : Mux  Inputs=22
  Mux6 : Mux  Inputs=6
  Sum{1..2,7,11..12} (5 alike) : Sum  Inputs=|++  SaturateOnIntegerOverflow=on  InputSameDT=on  OutDataTypeStr=Inherit: Same as first input
  Sum4 : Sum  SaturateOnIntegerOverflow=on  InputSameDT=on  OutDataTypeStr=Inherit: Same as first input
  Sum5 : Sum  Inputs=+-|  SaturateOnIntegerOverflow=on  InputSameDT=on  OutDataTypeStr=Inherit: Same as first input
  Sum6 : Sum  Inputs=++|  SaturateOnIntegerOverflow=on  InputSameDT=on  OutDataTypeStr=Inherit: Same as first input
  S : Outport  OutputWhenDisabled=reset  InitialOutput=0
  S_Modules : Outport  Port=2  OutputWhenDisabled=reset  InitialOutput=0
  wires:
  Mux1/1 -> S_Modules/1
  [M0_Sw] -> Mux1/2  "7~12"
  [M0_St] -> Mux1/1  "1~6"
  [M1_VAS] -> Mux1/3  "13"
  [M2_BFSH] -> Mux1/5  "15"
  [M2_VAS] -> Mux1/4  "14"
  [M6_GLU] -> Mux1/13  "23"
  [M6_HFL] -> Mux1/12  "22"
  [M4_HAM] -> Mux1/11  "21"
  [M4_GLU] -> Mux1/10  "20"
  [M4_HFL] -> Mux1/9  "19"
  [M3_HAM] -> Mux1/8  "18"
  [M3_GLU] -> Mux1/7  "17"
  [M3_HFL] -> Mux1/6  "16"
  [M10_VAS] -> Add3/4
  [M10_HFL] -> Add2/4
  [M9_HAM] -> Add1/3
  [M8_RF] -> Mux6/4
  [M8_BFSH] -> Add5/3
  [M9_BFSH] -> Add5/4
  [M7_BFSH] -> Add5/2
  [M6_HFL] -> Add2/3
  [M4_HAM] -> Add1/2
  [M4_HFL] -> Add2/2
  [M3_HAM] -> Add1/1
  [M3_HFL] -> Add2/1
  [M2_BFSH] -> Add5/1
  [M2_VAS] -> Add3/2
  [M1_VAS] -> Add3/1
  [M10_GLU] -> Add6/4
  [M6_GLU] -> Add6/3
  [M4_GLU] -> Add6/2
  [M3_GLU] -> Add6/1
  Demux17/3 -> [M10_VAS]  "VAS"
  Demux17/2 -> [M10_GLU]  "GLU"
  Demux17/1 -> [M10_HFL]  "HFL"
  Demux16/2 -> [M9_BFSH]  "BFSH"
  Demux16/1 -> [M9_HAM]  "HAM"
  Divide3/1 -> Demux17/1
  S_M10/1 -> Divide3/2
  Divide23/1 -> Demux16/1
  S_M9/1 -> Divide23/2
  Divide22/1 -> Demux5/1
  S_M8/1 -> Divide22/2
  Sum2/1 -> [M7_BFSH]  "M7_BFSH"
  S_M7_DS/1 -> Divide8/1
  Divide8/1 -> Divide21/2
  S_M7_Sw/1 -> Divide10/2
  Sum5/1 -> Divide15/2, Divide13/2
  Divide21/1 -> Sum2/2
  Sum12/1 -> [M6_GLU]  "M6_GLU"
  Sum11/1 -> [M6_HFL]  "M6_HFL"
  Divide19/1 -> Divide20/2
  Demux7/1 -> Sum11/1
  Demux6/2 -> Sum12/2
  Demux6/1 -> Sum11/2
  Divide20/1 -> Demux6/1
  Demux7/2 -> Sum12/1
  Divide9/1 -> Demux7/1
  S_M6/1 -> Divide19/1, Divide9/2
  Demux3/3 -> [M3_HAM]  "M3_HAM"
  Demux3/2 -> [M3_GLU]  "M3_GLU"
  Demux3/1 -> [M3_HFL]  "M3_HFL"
  Divide6/1 -> Demux3/1
  ILLoad/1 -> Divide6/3
  S_M3/1 -> Divide6/2
  Demux2/2 -> [M2_BFSH]  "M2_BFSH"
  Demux2/1 -> [M2_VAS]  "M2_VAS"
  Sum7/1 -> Demux2/1
  Divide17/1 -> Sum7/1
  S_M2/1 -> Divide15/1, Divide17/2  "VAS BFSH"
  Sum1/1 -> [M1_VAS]  "M1_VAS"
  Divide15/1 -> Divide16/2
  Divide16/1 -> Sum7/2
  Divide14/1 -> Sum1/2
  Divide13/1 -> Divide14/2
  Divide12/1 -> Sum1/1
  S_M1/1 -> Divide13/1, Divide12/2  "VAS"
  Divide4/1 -> [M0_St], Sum4/1
  Divide5/1 -> Sum4/2, [M0_Sw]
  S_0_St/1 -> Divide4/2
  S_0_Sw/1 -> Divide5/2
  Sum4/1 -> Sum6/1
  Sum6/1 -> S/1
  Mux6/1 -> Sum6/2
  Logical Operator6/1 -> Divide22/1, Divide23/1, Divide3/1, Divide10/1, Divide9/1, Divide5/1  "swing"
  Divide34/1 -> Divide8/2, Divide19/2
  Logical Operator7/1 -> Divide17/1, Divide12/1  "single stance"
  Divide7/1 -> Demux4/1
  Demux1/2 -> Divide34/1  "Tr_Sw"
  Add5/1 -> Mux6/6  "KFL"
  Add3/1 -> Mux6/5  "VAS"
  Demux4/3 -> [M4_HAM]  "M4_HAM"
  Add1/1 -> Mux6/3  "HAM"
  Demux4/2 -> [M4_GLU]  "M4_GLU"
  Add6/1 -> Mux6/2  "GLU"
  Add2/1 -> Mux6/1  "HFL"
  Demux4/1 -> [M4_HFL]  "M4_HFL"
  CLLoad/1 -> Divide34/2, Divide24/1
  Constant2/1 -> Sum5/1
  Divide24/1 -> Sum5/2
  Demux1/1 -> Divide24/2  "Tr_St_sup"
  Logical Operator1/1 -> Divide7/1  "Cswing"
  CStance/1 -> Logical Operator1/1
  S_M4/1 -> Divide7/2
  Logical Operator5/1 -> Logical Operator7/2
  ConI/1 -> Divide14/1, Divide16/1, Divide21/1, Divide20/1, Logical Operator5/1  "double stance"
  Stance/1 -> Divide6/1, Divide4/1, Logical Operator7/1, Logical Operator6/1  "stance"
  CtrlPar/1 -> Demux1/1
  [M8_VAS] -> Add3/3
  [M10_GLU] -> Mux1/21  "31"
  [M10_HFL] -> Mux1/20  "30"
  [M9_BFSH] -> Mux1/19  "29"
  [M9_HAM] -> Mux1/18  "28"
  [M8_BFSH] -> Mux1/17  "27"
  [M8_VAS] -> Mux1/16  "26"
  [M8_RF] -> Mux1/15  "25"
  [M7_BFSH] -> Mux1/14  "24"
  [M10_VAS] -> Mux1/22  "32"
  Divide10/1 -> Sum2/1
  Demux5/1 -> [M8_RF]  "RF"
  Demux5/3 -> [M8_BFSH]  "BFSH"
  Demux5/2 -> [M8_VAS]  "VAS"

== system atrias_boom_nmStand_fullCtrl/Control/Behavior Control/Virtual Neuromuscular Control/Neural Control Layer/L Swing Phase (sagittal) ==
  note: M10: prepare stance
  note: M9: stop leg
  note: M8: hold knee
  note: M7: flex knee
  note: M6: swing hip
  note: 0: Prestimulations
  note: Control During Stance -> Swing
  note: Left Swing Phase Control
  CtrlPar : Inport
  Stance : Inport  Port=2
  a_tgt : Inport  Port=3
  a : Inport  Port=4
  da : Inport  Port=5
  phiH : Inport  Port=6
  phiK : Inport  Port=7
  dphiK : Inport  Port=8
  l_clr : Inport  Port=9
  l : Inport  Port=10
  Enable : EnablePort  StatesWhenEnabling=reset
  Constant1 : Constant  Value=0  OutDataTypeStr=boolean
  Demux1 : Demux
  Divide{2..3,5,7..8} (5 alike) : Product
  Gain : Gain  Gain=-1
  Gain1 : Gain  Gain=-1
  Gain2 : Gain  Gain=-1
  Logical Operator : Logic  Operator=NOT  AllPortsSameDT=off  OutDataTypeStr=boolean
  Logical Operator1 : Logic  AllPortsSameDT=off  OutDataTypeStr=boolean
  Logical Operator2 : Logic  Operator=NOT  AllPortsSameDT=off  OutDataTypeStr=boolean
  Mux : Mux  Inputs=2
  Mux1 : Mux  Inputs=3
  Mux2 : Mux  Inputs=2
  Mux3 : Mux  Inputs=3
  Mux4 : Mux  Inputs=2
  Relational Operator : RelationalOperator  Operator=<=  OutDataTypeStr=boolean
  S-R Flip-Flop : simulink_extras/Flip Flops/S-R Flip-Flop  initial_condition=0
  Sum11 : Sum  Inputs=-+|  SaturateOnIntegerOverflow=on  InputSameDT=on  OutDataTypeStr=Inherit: Same as first input
  Sum6 : Sum  Inputs=|++  SaturateOnIntegerOverflow=on  InputSameDT=on  OutDataTypeStr=Inherit: Same as first input
  Sum7 : Sum  Inputs=|++  SaturateOnIntegerOverflow=on  InputSameDT=on  OutDataTypeStr=Inherit: Same as first input
  Terminator : Terminator
  kneei_flexion from alpha : Subsystem  TreatAsAtomicUnit=on
  kneeii_damp and hold &kneeiii_leg stop &kneeiv_stance preparation : Subsystem  TreatAsAtomicUnit=on
  negative half : Saturate  UpperLimit=0  LowerLimit=-inf  ZeroCross=off
  negative half2 : Saturate  UpperLimit=0  LowerLimit=-inf  ZeroCross=off
  negative half3 : Saturate  UpperLimit=0  LowerLimit=-inf  ZeroCross=off
  parSwH : Selector  InputPortWidth=Sw_i  Indices=parSwH_i
  parSwKi : Selector  InputPortWidth=Sw_i  Indices=parSwKi_i
  parSwPreS : Selector  InputPortWidth=Sw_i  Indices=parSwPreS_i
  positive half1 : Saturate  UpperLimit=inf  LowerLimit=0  ZeroCross=off
  positive half2 : Saturate  UpperLimit=inf  LowerLimit=0  ZeroCross=off
  S_Sw_0 : Outport  OutputWhenDisabled=reset  InitialOutput=0
  S_M6 [HFL GLU] : Outport  Port=2  OutputWhenDisabled=reset  InitialOutput=0
  S_M7_DS [BFSH] : Outport  Port=3  OutputWhenDisabled=reset  InitialOutput=0
  S_M7_Sw [VAS BFSH] : Outport  Port=4  OutputWhenDisabled=reset  InitialOutput=0
  M8 [RF VAS BFSH] : Outport  Port=5  OutputWhenDisabled=reset  InitialOutput=0
  M9 [HAM BFSH] : Outport  Port=6  OutputWhenDisabled=reset  InitialOutput=0
  M10 [HFL GLU VAS] : Outport  Port=7  OutputWhenDisabled=reset  InitialOutput=0
  Phase [M7 M8 M9 M10] : Outport  Port=8  OutputWhenDisabled=reset  InitialOutput=0
  wires:
  phiH/1 -> kneeii_damp and hold &kneeiii_leg stop &kneeiv_stance preparation/5(phiH)
  phiK/1 -> kneeii_damp and hold &kneeiii_leg stop &kneeiv_stance preparation/6(phiK)
  dphiK/1 -> kneeii_damp and hold &kneeiii_leg stop &kneeiv_stance preparation/7(dphiK)
  Gain2/1 -> negative half2/1
  da/1 -> kneeii_damp and hold &kneeiii_leg stop &kneeiv_stance preparation/4(da), negative half3/1, Gain2/1, negative half/1
  l_clr/1 -> Relational Operator/2
  l/1 -> Relational Operator/1
  Sum11/1 -> Gain/1, positive half2/1  "del_alp"
  a/1 -> Sum11/2, kneeii_damp and hold &kneeiii_leg stop &kneeiv_stance preparation/3(a)
  kneeii_damp and hold &kneeiii_leg stop &kneeiv_stance preparation/1(phase [M8 M9 M10]) -> Mux/2
  Mux/1 -> Phase [M7 M8 M9 M10]/1
  Divide8/1 -> Sum7/2
  Sum7/1 -> Mux2/2  "GLU"
  Divide2/1 -> Sum7/1  "GLU"
  negative half2/1 -> Divide8/2
  negative half3/1 -> Divide7/2
  Sum6/1 -> Mux2/1  "HFL"
  Divide7/1 -> Sum6/2
  Divide5/1 -> Sum6/1  "HFL"
  Demux1/4 -> Divide8/1  "Sw_dalpGain_GLU"
  Demux1/2 -> Divide7/1  "Sw_dalpGain_HFL"
  Mux1/1 -> M10 [HFL GLU VAS]/1
  Mux4/1 -> M9 [HAM BFSH]/1
  Mux3/1 -> M8 [RF VAS BFSH]/1
  Mux2/1 -> S_M6 [HFL GLU]/1
  kneeii_damp and hold &kneeiii_leg stop &kneeiv_stance preparation/9(SVAS_Sw_kiv) -> Mux1/3  "VAS"
  kneeii_damp and hold &kneeiii_leg stop &kneeiv_stance preparation/5(SHAM_Sw_kiii) -> Mux4/1  "HAM"
  parSwPreS/1 -> S_Sw_0/1
  Logical Operator2/1 -> Logical Operator1/1
  Stance/1 -> Logical Operator2/1
  Relational Operator/1 -> Logical Operator1/2
  Logical Operator1/1 -> S-R Flip-Flop/1
  kneeii_damp and hold &kneeiii_leg stop &kneeiv_stance preparation/6(SBFSH_Sw_kiii) -> Mux4/2  "BFSH"
  kneeii_damp and hold &kneeiii_leg stop &kneeiv_stance preparation/8(SGLU_Sw_kiv) -> Mux1/2  "GLU"
  kneeii_damp and hold &kneeiii_leg stop &kneeiv_stance preparation/7(SHFL_Sw_kiv) -> Mux1/1  "HFL"
  Logical Operator/1 -> kneei_flexion from alpha/Enable, Mux/1
  S-R Flip-Flop/1 -> Logical Operator/1, kneeii_damp and hold &kneeiii_leg stop &kneeiv_stance preparation/Enable
  S-R Flip-Flop/2 -> Terminator/1
  Constant1/1 -> S-R Flip-Flop/2
  Divide3/1 -> kneei_flexion from alpha/1(SBFSH), S_M7_DS [BFSH]/1  "BFSH"
  negative half/1 -> Gain1/1
  Gain1/1 -> Divide3/1
  Demux1/3 -> Divide2/1  "Sw_alpGain_GLU"
  positive half1/1 -> Divide2/2
  Gain/1 -> positive half1/1
  Demux1/1 -> Divide5/1  "Sw_alpGain_HFL"
  positive half2/1 -> Divide5/2  "del_alp"
  a_tgt/1 -> Sum11/1, kneeii_damp and hold &kneeiii_leg stop &kneeiv_stance preparation/2(a_tgt)
  parSwH/1 -> Demux1/1
  CtrlPar/1 -> parSwH/1, kneeii_damp and hold &kneeiii_leg stop &kneeiv_stance preparation/1(CtrlPar), parSwKi/1, parSwPreS/1
  parSwKi/1 -> Divide3/2  "Sw_dalpGain_BFSH"
  kneei_flexion from alpha/1(SBFSH_Sw_ki) -> S_M7_Sw [VAS BFSH]/1
  kneeii_damp and hold &kneeiii_leg stop &kneeiv_stance preparation/2(SRF_Sw_kii) -> Mux3/1  "RF"
  kneeii_damp and hold &kneeiii_leg stop &kneeiv_stance preparation/3(SVAS_Sw_kii) -> Mux3/2  "VAS"
  kneeii_damp and hold &kneeiii_leg stop &kneeiv_stance preparation/4(SBFSH_Sw_kii) -> Mux3/3  "BFSH"
